simulink model "motorlagleadcompensatorPushingValuesToWorkspaceForManipulation"  (R2021b)
settings: Solver=VariableStepAuto  StartTime=0.0  StopTime=5  RelTol=1e-3
values from neighbouring files (symbols this model uses):
  b = 0.1    [simscapeParameters.m]    (also in simscapeVisualization.m)
  J = 0.01    [simscapeParameters.m]    (also in simscapeVisualization.m)
  K = 0.01    [simscapeParameters.m]    (also in simscapeVisualization.m)
  L = 0.5    [simscapeParameters.m]    (also in simscapeVisualization.m)
  R = 1    [simscapeParameters.m]    (also in simscapeVisualization.m)
settings Model: Creator=Joshua  LastModifiedBy=Joshua

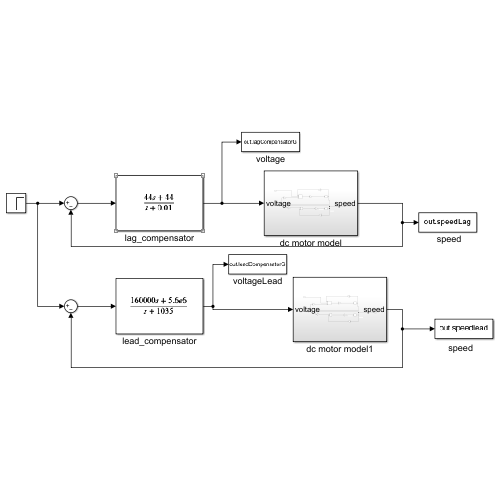
[thumbnail: Simulink's stored preview of the top-level diagram]
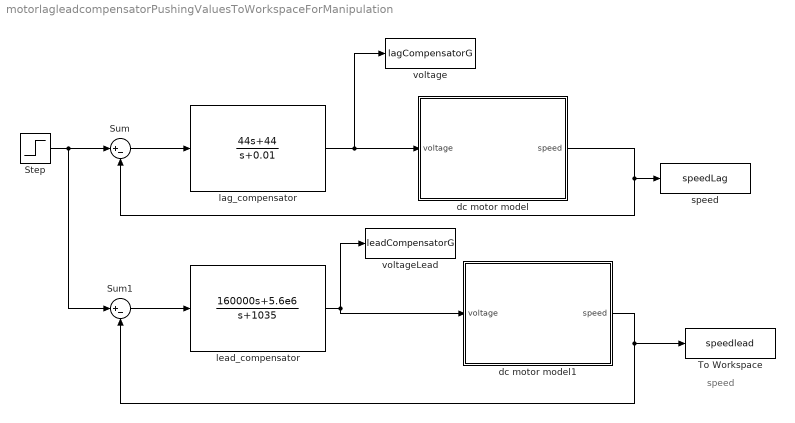
== system motorlagleadcompensatorPushingValuesToWorkspaceForManipulation ==
  note: speed
  " speed" : ToWorkspace  VariableName=speedLag  SampleTime=-1
  Step : Step  SampleTime=0
  Sum : Sum  Inputs=|+-
  Sum1 : Sum  Inputs=|+-
  To Workspace : ToWorkspace  VariableName=speedlead  SampleTime=-1
  dc motor model : Subsystem
  dc motor model1 : Subsystem
  lag_compensator : TransferFcn  Numerator=[44 44]  Denominator=[1 0.01]
  lead_compensator : TransferFcn  Numerator=[160000 5.6e6]  Denominator=[1 1035]
  voltage : ToWorkspace  VariableName=lagCompensatorG  SampleTime=-1
  voltageLead : ToWorkspace  VariableName=leadCompensatorG  SampleTime=-1
  wires:
  lead_compensator/1 -> dc motor model1/1(voltage), voltageLead/1
  Step/1 -> Sum1/1, Sum/1
  lag_compensator/1 -> voltage/1, dc motor model/1(voltage)
  Sum1/1 -> lead_compensator/1
  dc motor model1/1(speed) -> Sum1/2, To Workspace/1
  dc motor model/1(speed) -> Sum/2, " speed"/1
  Sum/1 -> lag_compensator/1

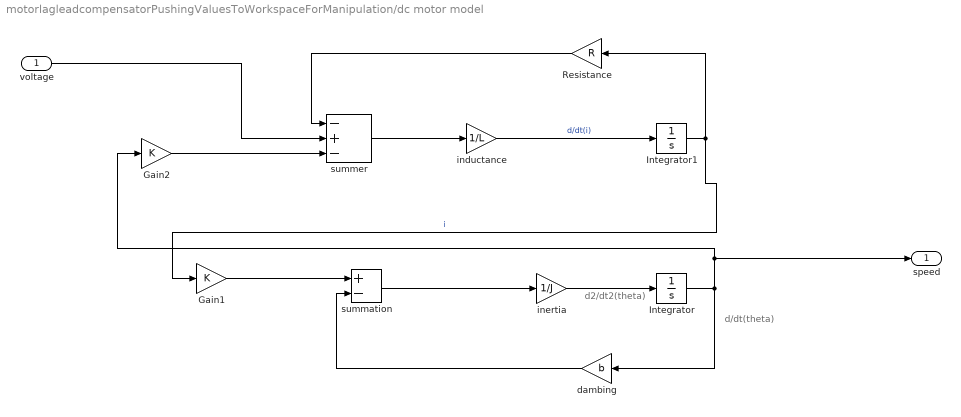
== system motorlagleadcompensatorPushingValuesToWorkspaceForManipulation/dc motor model ==
  note: d/dt(theta)
  note: d2/dt2(theta)
  voltage : Inport
  Gain1 : Gain  Gain=K
  Gain2 : Gain  Gain=K
  Integrator : Integrator
  Integrator1 : Integrator
  Resistance : Gain  Gain=R
  dambing : Gain  Gain=b
  inductance : Gain  Gain=1/L
  inertia : Gain  Gain=1/J
  summation : Sum  Inputs=+-
  summer : Sum  Inputs=-+-
  speed : Outport
  wires:
  inductance/1 -> Integrator1/1  "d/dt(i)"
  Integrator1/1 -> Gain1/1, Resistance/1  "i"
  summer/1 -> inductance/1
  summation/1 -> inertia/1
  dambing/1 -> summation/2
  Gain1/1 -> summation/1
  Integrator/1 -> speed/1, Gain2/1, dambing/1
  voltage/1 -> summer/2
  inertia/1 -> Integrator/1
  Resistance/1 -> summer/1
  Gain2/1 -> summer/3

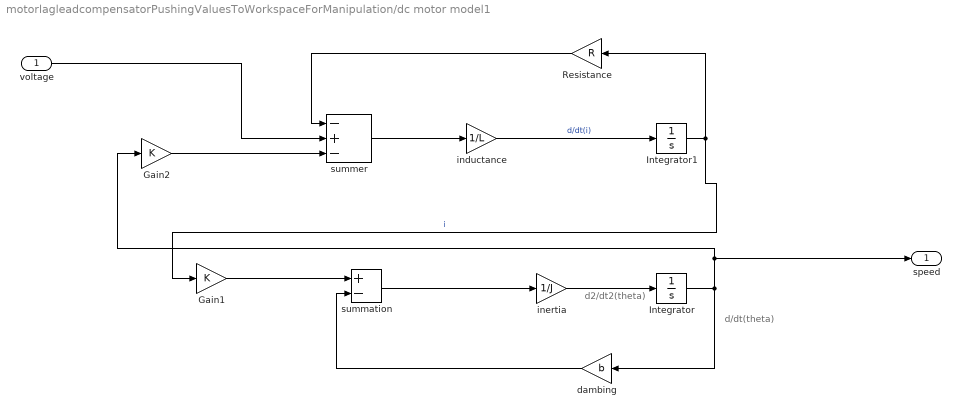
== system motorlagleadcompensatorPushingValuesToWorkspaceForManipulation/dc motor model1 ==
  note: d/dt(theta)
  note: d2/dt2(theta)
  voltage : Inport
  Gain1 : Gain  Gain=K
  Gain2 : Gain  Gain=K
  Integrator : Integrator
  Integrator1 : Integrator
  Resistance : Gain  Gain=R
  dambing : Gain  Gain=b
  inductance : Gain  Gain=1/L
  inertia : Gain  Gain=1/J
  summation : Sum  Inputs=+-
  summer : Sum  Inputs=-+-
  speed : Outport
  wires:
  inductance/1 -> Integrator1/1  "d/dt(i)"
  Integrator1/1 -> Gain1/1, Resistance/1  "i"
  summer/1 -> inductance/1
  summation/1 -> inertia/1
  dambing/1 -> summation/2
  Gain1/1 -> summation/1
  Integrator/1 -> speed/1, Gain2/1, dambing/1
  voltage/1 -> summer/2
  inertia/1 -> Integrator/1
  Resistance/1 -> summer/1
  Gain2/1 -> summer/3
